simulink model "lab5_2"  (R2021b)
settings: Solver=VariableStepAuto  StartTime=0.0  StopTime=50  MaxStep=0.01  RelTol=1e-3
libraries: simulink_extras x2
settings Model: Creator=asr77  LastModifiedBy=asr77

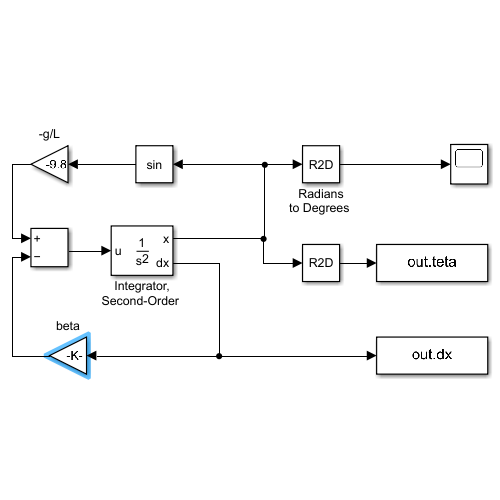
[thumbnail: Simulink's stored preview of the top-level diagram]
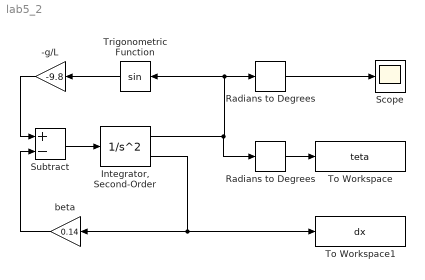
== system lab5_2 ==
  -g/L : Gain  Gain=-9.8
  "Integrator, Second-Order " : SecondOrderIntegrator  ICX=2*pi/3+0.01  ICDXDT=0
  Radians to Degrees : simulink_extras/Transformations/Radians to Degrees
  "Radians to Degrees " : simulink_extras/Transformations/Radians to Degrees
  Scope : Scope
  Subtract : Sum  Inputs=+-
  To Workspace : ToWorkspace  VariableName=teta  SaveFormat=Timeseries  SampleTime=-1
      settings: Save2DSignal=2-D array (concatenate along first dimension)
  To Workspace1 : ToWorkspace  VariableName=dx  SaveFormat=Timeseries  SampleTime=-1
  Trigonometric Function : Trigonometry
  beta : Gain  Gain=0.14
  wires:
  "Integrator, Second-Order "/1 -> Radians to Degrees/1, Trigonometric Function/1, "Radians to Degrees "/1
  -g/L/1 -> Subtract/1
  "Radians to Degrees "/1 -> Scope/1
  "Integrator, Second-Order "/2 -> To Workspace1/1, beta/1
  Subtract/1 -> "Integrator, Second-Order "/1
  Radians to Degrees/1 -> To Workspace/1
  beta/1 -> Subtract/2
  Trigonometric Function/1 -> -g/L/1
